simulink subsystem "Limelight_Tag_Corrections_sub"  (R2023b)
settings: Solver=VariableStepAuto  StartTime=0.0  StopTime=10.0  RelTol=1e-3
undefined symbols (not defined in the file): Limelight_Tag_Angle_Offset, Limelight_Tag_X_Offset, Limelight_Tag_Y_Offset
settings Model: Creator=ander  LastModifiedBy=ander

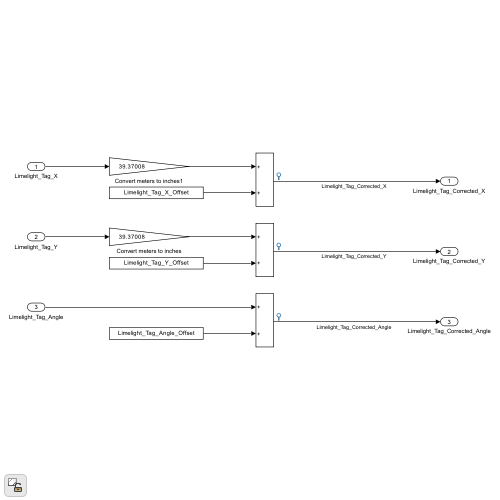
[thumbnail: Simulink's stored preview of the top-level diagram]
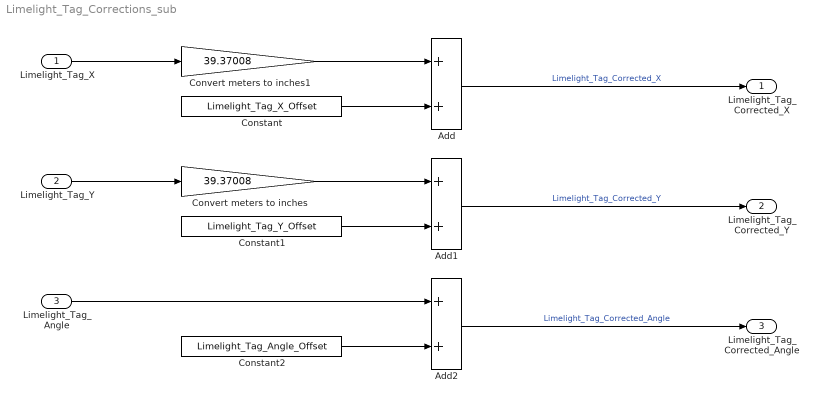
== system Limelight_Tag_Corrections_sub ==
  Limelight_Tag_X : Inport
  Limelight_Tag_Y : Inport  Port=2
  Limelight_Tag_Angle : Inport  Port=3
  Add : Sum
  Add1 : Sum
  Add2 : Sum
  Constant : Constant  Value=Limelight_Tag_X_Offset
  Constant1 : Constant  Value=Limelight_Tag_Y_Offset
  Constant2 : Constant  Value=Limelight_Tag_Angle_Offset
  Convert meters to inches : Gain  Gain=39.37008
  Convert meters to inches1 : Gain  Gain=39.37008
  Limelight_Tag_Corrected_X : Outport
  Limelight_Tag_Corrected_Y : Outport  Port=2
  Limelight_Tag_Corrected_Angle : Outport  Port=3
  wires:
  Limelight_Tag_X/1 -> Convert meters to inches1/1
  Constant/1 -> Add/2
  Add/1 -> Limelight_Tag_Corrected_X/1  "Limelight_Tag_Corrected_X"
  Constant1/1 -> Add1/2
  Constant2/1 -> Add2/2
  Limelight_Tag_Angle/1 -> Add2/1
  Limelight_Tag_Y/1 -> Convert meters to inches/1
  Add1/1 -> Limelight_Tag_Corrected_Y/1  "Limelight_Tag_Corrected_Y"
  Add2/1 -> Limelight_Tag_Corrected_Angle/1  "Limelight_Tag_Corrected_Angle"
  Convert meters to inches/1 -> Add1/1
  Convert meters to inches1/1 -> Add/1
